simulink model "Passive_cell_Balancing"  (R2023a)
settings: Solver=VariableStepAuto  StartTime=0.0  StopTime=10  RelTol=1e-3
undefined symbols (not defined in the file): Ion, Lithium
libraries: spsBatteryLib x3, spsIdealSwitchLib x3, spsSeriesRLCLoadLib x3, spsVoltageMeasurementLib x1, sps_lib x1
settings Model: Creator=matha  LastModifiedBy=matha

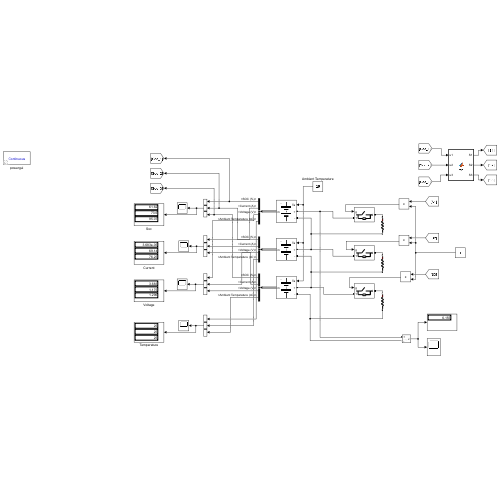
[thumbnail: Simulink's stored preview of the top-level diagram]
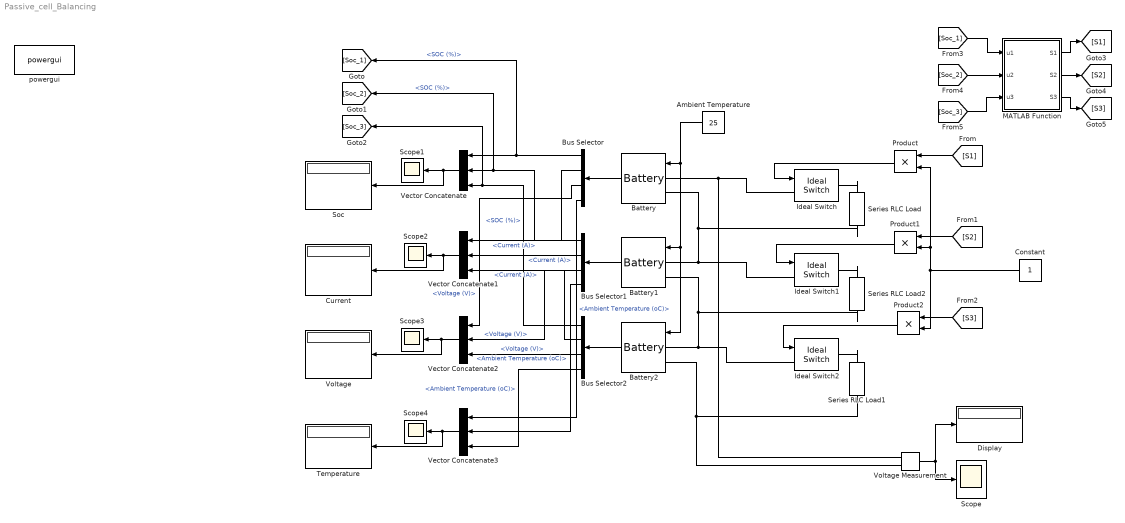
== system Passive_cell_Balancing ==
  Ambient Temperature : Constant  Value=25
  Battery : spsBatteryLib/Battery  BatType=Lithium-Ion  ShowTempParam=on  ThermalPreset="3.6V  4.5Ah"  ShowAgeParam=on  NomV=3.3  NomQ=4.5  SOC=65  Batt_Tr=1  PresetModel=off  MaxQ=4.8  MinV=2.475  FullV=4.1  Dis_rate=0.9  R=0.00756  Normal_OP=4.0696  expZone="[3.88         0.5]"  current=[6.5 13 32.5]  Units=Time  Tci=20  NomT=115  T2=0  MaxQ2=4.2  FullV2=4  Normal_OP2=3.1  expZone2="[3.8        0.25]"  Rca=0.06  ti=1000  Dp=0  Neq0=0  Tsim=1e6  Ta1=25  Qeol=5.4*0.9  Reol=0.013333*1.2  Char_age=[2.3478, 3]  Dis_age=[2.3478, 10]  N1=1500  N2=10500  N3=1000  N4=1400  Ta2=45  N5=950
  Battery1 : spsBatteryLib/Battery  BatType=Lithium-Ion  ShowTempParam=on  ThermalPreset="3.6V  4.5Ah"  ShowAgeParam=on  NomV=3.3  NomQ=4.5  SOC=80  Batt_Tr=1  PresetModel=off  MaxQ=4.8  MinV=2.475  FullV=4.1  Dis_rate=0.9  R=0.00756  Normal_OP=4.0696  expZone="[3.88         0.5]"  current=[6.5 13 32.5]  Units=Time  Tci=20  NomT=115  T2=0  MaxQ2=4.2  FullV2=4  Normal_OP2=3.1  expZone2="[3.8        0.25]"  Rca=0.06  ti=1000  Dp=0  Neq0=0  Tsim=1e6  Ta1=25  Qeol=5.4*0.9  Reol=0.013333*1.2  Char_age=[2.3478, 3]  Dis_age=[2.3478, 10]  N1=1500  N2=10500  N3=1000  N4=1400  Ta2=45  N5=950
  Battery2 : spsBatteryLib/Battery  BatType=Lithium-Ion  ShowTempParam=on  ThermalPreset="3.6V  4.5Ah"  ShowAgeParam=on  NomV=3.3  NomQ=4.5  SOC=100  Batt_Tr=1  PresetModel=off  MaxQ=4.8  MinV=2.475  FullV=4.1  Dis_rate=0.9  R=0.00756  Normal_OP=4.0696  expZone="[3.88         0.5]"  current=[6.5 13 32.5]  Units=Time  Tci=20  NomT=115  T2=0  MaxQ2=4.2  FullV2=4  Normal_OP2=3.1  expZone2="[3.8        0.25]"  Rca=0.06  ti=1000  Dp=0  Neq0=0  Tsim=1e6  Ta1=25  Qeol=5.4*0.9  Reol=0.013333*1.2  Char_age=[2.3478, 3]  Dis_age=[2.3478, 10]  N1=1500  N2=10500  N3=1000  N4=1400  Ta2=45  N5=950
  Bus Selector : BusSelector  OutputSignals=SOC (%),Current (A),Voltage (V),Ambient Temperature (oC)
  Bus Selector1 : BusSelector  OutputSignals=SOC (%),Current (A),Voltage (V),Ambient Temperature (oC)
  Bus Selector2 : BusSelector  OutputSignals=SOC (%),Current (A),Voltage (V),Ambient Temperature (oC)
  Constant : Constant
  Current : Display
  Display : Display
  Ideal Switch : spsIdealSwitchLib/Ideal Switch  Ron=0.001  Lon=0  IC=0  Rs=1e5  Cs=inf  Measurements=off
  Ideal Switch1 : spsIdealSwitchLib/Ideal Switch  Ron=0.001  Lon=0  IC=0  Rs=1e5  Cs=inf  Measurements=off
  Ideal Switch2 : spsIdealSwitchLib/Ideal Switch  Ron=0.001  Lon=0  IC=0  Rs=1e5  Cs=inf  Measurements=off
  MATLAB Function : MATLAB Function  TreatAsAtomicUnit=on
  Product : Product
  Product1 : Product
  Product2 : Product
  Scope{,1..4} (5 alike) : Scope
  Series RLC Load : spsSeriesRLCLoadLib/Series RLC Load  LConnTagsString=a  RConnTagsString=__new0  NominalVoltage=4  NominalFrequency=0.1  ActivePower=1000  InductivePower=0  CapacitivePower=0  Setx0=off  InitialVoltage=0  SetiL0=off  InitialCurrent=0  Measurements=None  LoadType=constant Z
  Series RLC Load1 : spsSeriesRLCLoadLib/Series RLC Load  LConnTagsString=a  RConnTagsString=__new0  NominalVoltage=4  NominalFrequency=0.1  ActivePower=1000  InductivePower=0  CapacitivePower=0  Setx0=off  InitialVoltage=0  SetiL0=off  InitialCurrent=0  Measurements=None  LoadType=constant Z
  Series RLC Load2 : spsSeriesRLCLoadLib/Series RLC Load  LConnTagsString=a  RConnTagsString=__new0  NominalVoltage=4  NominalFrequency=0.1  ActivePower=1000  InductivePower=0  CapacitivePower=0  Setx0=off  InitialVoltage=0  SetiL0=off  InitialCurrent=0  Measurements=None  LoadType=constant Z
  Soc : Display
  Temperature : Display
  Vector Concatenate{,1..3} (4 alike) : Concatenate  NumInputs=3
  Voltage : Display
  Voltage Measurement : spsVoltageMeasurementLib/Voltage Measurement  PhasorSimulation=off  OutputType=Complex  PSBequivalent=0
  powergui : sps_lib/powergui  Priority=1  SimulationMode=Continuous  SampleTime=50e-6  frequency=60  Iterations=50  frequencyindice=0  Pbase=100e6  ErrMax=1e-4  UnitsV=kV  UnitsW=MW  buscounter=0  FunctionMessages=off  echomessages=off  EnableUseOfTLC=off  CurrentSourceSwitches=off  DisableSnubberDevices=off  DisableRonSwitches=off  DisableVfSwitches=off  DisplayEquations=off  AutomaticDiscreteSolvers=off  SolverType=Tustin/Backward Euler (TBE)  Interpol=off  ExternalGateDelay=off  methode=off  Ts=100  x0status=blocks  SPID=on  SwTol=0  HookPort=off  NonlinearTolerance=1e-4  nMaxIteration=100  ContinueOnMaxIteration=off  RestoreLinks=warning  ResistiveCurrentMeasurement=off  Frange=[0:2:500]  Ylog=off  Xlog=on  ShowGrid=off  save=off  variable=ZData  structure=0  ZoomFFT=off  StartTime=0.0  cycles=1  DisplayStyle=1  fundamental=60  FreqAxis=off  MaxFrequency=1000  frequencyindicesteady=1  RmsSteady=1  display=off
  wires:
  Ambient Temperature/1 -> Battery2/1, Battery1/1, Battery/1
  Voltage Measurement/1 -> Display/1, Scope/1
  Product/1 -> Ideal Switch/1
  Product1/1 -> Ideal Switch1/1
  Product2/1 -> Ideal Switch2/1
  [S1] -> Product/1
  [S3] -> Product2/1
  [S2] -> Product1/1
  Constant/1 -> Product/2, Product1/2, Product2/2
  Battery/1 -> Bus Selector/1
  Battery2/1 -> Bus Selector2/1
  Battery1/1 -> Bus Selector1/1
  Bus Selector/1 -> [Soc_1], Vector Concatenate/1  "<SOC (%)>"
  Bus Selector1/1 -> [Soc_2], Vector Concatenate/2  "<SOC (%)>"
  Bus Selector2/1 -> [Soc_3], Vector Concatenate/3  "<SOC (%)>"
  Bus Selector/2 -> Vector Concatenate1/1  "<Current (A)>"
  Bus Selector1/2 -> Vector Concatenate1/2  "<Current (A)>"
  Bus Selector2/2 -> Vector Concatenate1/3  "<Current (A)>"
  Bus Selector/3 -> Vector Concatenate2/1  "<Voltage (V)>"
  Bus Selector1/3 -> Vector Concatenate2/2  "<Voltage (V)>"
  Bus Selector2/3 -> Vector Concatenate2/3  "<Voltage (V)>"
  Vector Concatenate/1 -> Soc/1, Scope1/1
  Vector Concatenate1/1 -> Current/1, Scope2/1
  Vector Concatenate2/1 -> Scope3/1, Voltage/1
  Vector Concatenate3/1 -> Temperature/1, Scope4/1
  Bus Selector/4 -> Vector Concatenate3/1  "<Ambient Temperature (oC)>"
  Bus Selector1/4 -> Vector Concatenate3/2  "<Ambient Temperature (oC)>"
  Bus Selector2/4 -> Vector Concatenate3/3  "<Ambient Temperature (oC)>"
  [Soc_1] -> MATLAB Function/1(u1)
  [Soc_2] -> MATLAB Function/2(u2)
  [Soc_3] -> MATLAB Function/3(u3)
  MATLAB Function/1(S1) -> [S1]
  MATLAB Function/2(S2) -> [S2]
  MATLAB Function/3(S3) -> [S3]
  connections:
  Battery/LConn2 -- Ideal Switch1/LConn1 -- Battery1/LConn1 -- Series RLC Load/RConn1
  Battery1/LConn2 -- Ideal Switch2/LConn1 -- Battery2/LConn1 -- Series RLC Load2/RConn1
  Ideal Switch/LConn1 -- Voltage Measurement/LConn1 -- Battery/LConn1
  Series RLC Load/LConn1 -- Ideal Switch/RConn1
  Series RLC Load2/LConn1 -- Ideal Switch1/RConn1
  Series RLC Load1/LConn1 -- Ideal Switch2/RConn1
  Series RLC Load1/RConn1 -- Voltage Measurement/LConn2 -- Battery2/LConn2

== matlab function Passive_cell_Balancing/MATLAB Function ==
  data: u1 input; S1 output; u2 input; u3 input; S2 output; S3 output
function [S1,S2,S3] = fcn(u1,u2,u3)

% u1 = double(u1);
% u2 = double(u2);
% u3 = double(u3);

if ((u1>u2) || (u1>u3)) 
    S1 = 1;
else
    S1 = 0;
end

if ((u2>u1) || (u2>u3))
    S2 = 1;
else
    S2 = 0;
end

    if ((u3>u1) || (u3>u2))
        S3 = 1;
    else
        S3 = 0;
    end
